simulink model "Simple_2_DPRAM_test"  (R2019b)
settings: Solver=FixedStepAuto  StartTime=0.0  StopTime=stop_time  RelTol=1e-3
InitFcn:
  | init;
StopFcn:
  | % save timeseries things as actual useful data.
values from neighbouring files (symbols this model uses):
  Addr_Bits = 4    [init.m]
  RAM_0_SEL = 0    [init.m]
  RAM_1_SEL = 1    [init.m]
  Sel_Bits = 2    [init.m]
  Ts = 1/Fs    (= 2.08333333333e-05)    [init.m]
  Ts_system = 1/Fs_system    (= 2e-08)    [init.m]
libraries: hdlsllib x7, simulink x5
settings Model: Creator=Balad  LastModifiedBy=Balad
settings SFSimCC: CustomCodeUndefinedFunction=UseInterfaceOnly

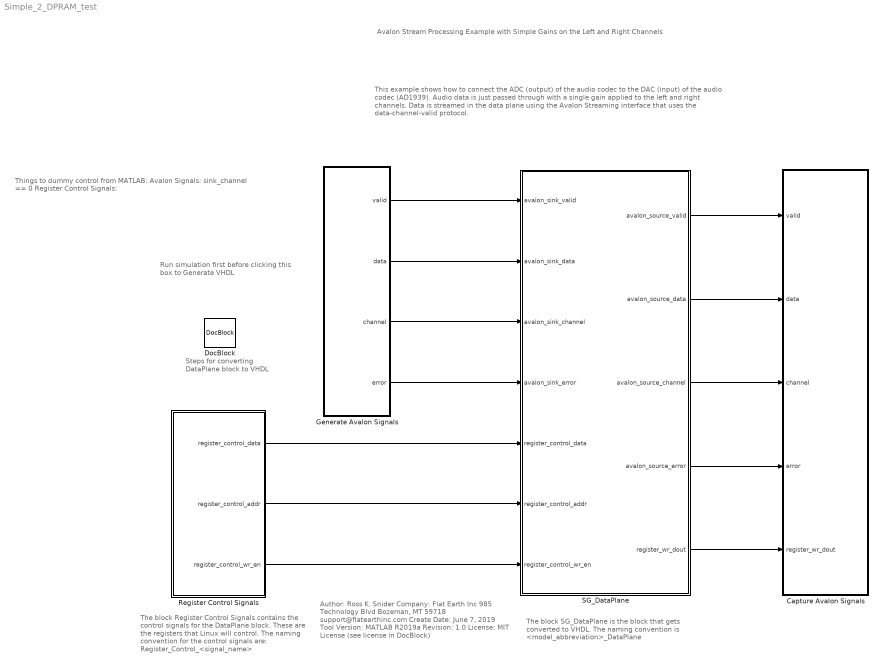
== system Simple_2_DPRAM_test ==
  note: Avalon Stream Processing Example
      | with Simple Gains on the Left and Right Channels
  note: The block SG_DataPlane is the block that gets
      | converted to VHDL. The naming convention is
      | <model_abbreviation>_DataPlane
  note: This example shows how to connect the ADC (output) of the audio codec to the DAC (input) of the audio codec (AD1939). Audio data is just passed through with a single gain applied to the left and right channels. Data is streamed in the data plane using the Avalon Streaming interface that uses the data-channel-valid protocol.
  note: The block Register Control Signals contains
      | the control signals for the DataPlane block.
      | These are the registers that Linux will control.
      | The naming convention for the control
      | signals are:  Register_Control_<signal_name>
  note: Author:          Ross K. Snider
      | Company:     Flat Earth Inc
      |                       985 Technology Blvd
      |                       Bozeman, MT 59718
      |                       support@flatearthinc.com
      | Create Date:  June 7, 2019
      | Tool Version:  MATLAB R2019a
      | Revision:        1.0
      | License:          MIT License (see license in DocBlock)
  note: Run simulation first
      | before clicking this box to
      | Generate VHDL
  note: Steps for converting
      | DataPlane block
      | to VHDL
  note: Things to dummy control from MATLAB:
      | Avalon Signals:
      | sink_channel == 0
      | Register Control Signals:
  Capture Avalon Signals : Subsystem
  DocBlock : simulink/Model-Wide Utilities/DocBlock  DocumentType=HTML
      content=|
      | <html><head></head><body>
      | Type your documentation here</body></html>
  Generate Avalon Signals : Subsystem
  Register Control Signals : Subsystem
  SG_DataPlane : Subsystem  TreatAsAtomicUnit=on
  wires:
  SG_DataPlane/2(avalon_source_data) -> Capture Avalon Signals/2(data)
  Generate Avalon Signals/1(valid) -> SG_DataPlane/1(avalon_sink_valid)
  Generate Avalon Signals/2(data) -> SG_DataPlane/2(avalon_sink_data)
  Register Control Signals/2(register_control_addr) -> SG_DataPlane/6(register_control_addr)
  SG_DataPlane/1(avalon_source_valid) -> Capture Avalon Signals/1(valid)
  SG_DataPlane/4(avalon_source_error) -> Capture Avalon Signals/4(error)
  Generate Avalon Signals/4(error) -> SG_DataPlane/4(avalon_sink_error)
  Register Control Signals/1(register_control_data) -> SG_DataPlane/5(register_control_data)
  SG_DataPlane/3(avalon_source_channel) -> Capture Avalon Signals/3(channel)
  Generate Avalon Signals/3(channel) -> SG_DataPlane/3(avalon_sink_channel)
  Register Control Signals/3("register_control_wr_en ") -> SG_DataPlane/7("register_control_wr_en ")
  SG_DataPlane/5(register_wr_dout) -> Capture Avalon Signals/5(register_wr_dout)

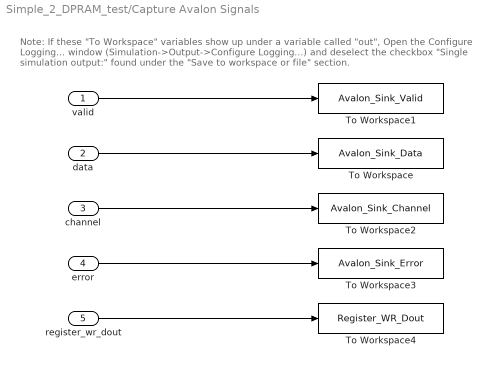
== system Simple_2_DPRAM_test/Capture Avalon Signals ==
  note: Note:  If these "To Workspace" variables show up under a variable called "out",
      | Open the Configure Logging... window (Simulation->Output->Configure Logging...)
      | and deselect the checkbox "Single simulation output:" found under the "Save to workspace or file" section.
  valid : Inport
  data : Inport  Port=2
  channel : Inport  Port=3
  error : Inport  Port=4
  register_wr_dout : Inport  Port=5
  To Workspace : ToWorkspace  VariableName=Avalon_Sink_Data  SaveFormat=Timeseries  SampleTime=-1
  To Workspace1 : ToWorkspace  VariableName=Avalon_Sink_Valid  SaveFormat=Timeseries  SampleTime=-1
  To Workspace2 : ToWorkspace  VariableName=Avalon_Sink_Channel  SaveFormat=Timeseries  SampleTime=-1
  To Workspace3 : ToWorkspace  VariableName=Avalon_Sink_Error  SaveFormat=Timeseries  SampleTime=-1
  To Workspace4 : ToWorkspace  VariableName=Register_WR_Dout  SaveFormat=Timeseries  SampleTime=-1
  wires:
  data/1 -> To Workspace/1
  valid/1 -> To Workspace1/1
  error/1 -> To Workspace3/1
  channel/1 -> To Workspace2/1
  register_wr_dout/1 -> To Workspace4/1

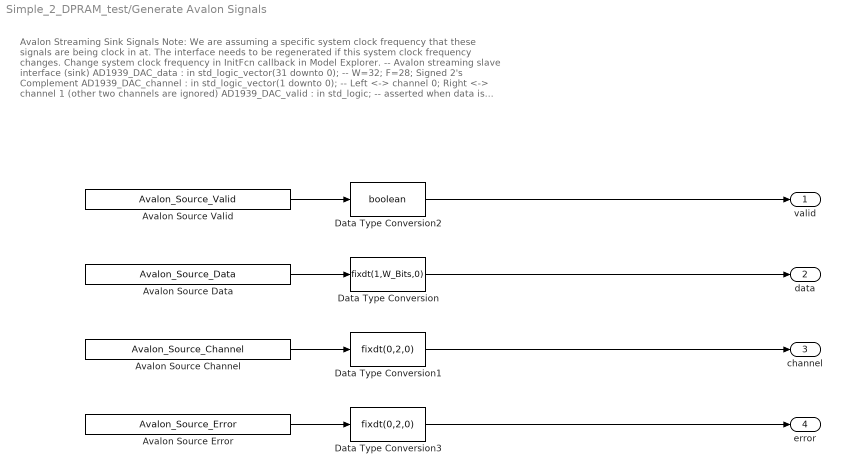
== system Simple_2_DPRAM_test/Generate Avalon Signals ==
  note: Avalon Streaming Sink Signals
      | Note: We are assuming a specific system clock frequency that these signals are being clock in at.
      | The interface needs to be regenerated if this system clock frequency changes. Change system clock frequency in InitFcn callback in Model Explorer.
      |
      | -- Avalon streaming slave interface (sink)
      | AD1939_DAC_data : in std_logic_vector(31 downto 0); -- W=32; F=28; Signed 2's Complement
      | AD1939_DAC_channel : in std_logic_vector(1 downto 0); -- Left <-> channel 0; Right <-> channel 1 (other two channels are ignored)
      | AD1939_DAC_valid : in std_logic; -- asserted when data is valid
      | AD1939_DAC_error : in std_logic_vector(1 downto 0) -- error channel is ignored, assumed to be error free at this point
      |
      | For more information on the data-channel-valid protocol, see chapter 5 in Intel's Avalon Interfaced Specification (p. 40) at https://www.intel.com/content/dam/www/programmable/us/en/pdfs/literature/manual/mnl_avalon_spec.pdf
  Avalon Source Channel : FromWorkspace  VariableName=Avalon_Source_Channel  SampleTime=Ts_system  Interpolate=off  OutputAfterFinalValue=Holding final value
  "Avalon Source Data " : FromWorkspace  VariableName=Avalon_Source_Data  SampleTime=Ts_system  Interpolate=off  OutputAfterFinalValue=Holding final value
  Avalon Source Error : FromWorkspace  VariableName=Avalon_Source_Error  SampleTime=Ts_system  Interpolate=off  OutputAfterFinalValue=Holding final value
  Avalon Source Valid : FromWorkspace  VariableName=Avalon_Source_Valid  SampleTime=Ts_system  Interpolate=off  OutputAfterFinalValue=Holding final value
  Data Type Conversion : DataTypeConversion  OutDataTypeStr=fixdt(1,W_Bits,0)
  Data Type Conversion1 : DataTypeConversion  OutDataTypeStr=fixdt(0,2,0)
  Data Type Conversion2 : DataTypeConversion  OutDataTypeStr=boolean
  Data Type Conversion3 : DataTypeConversion  OutDataTypeStr=fixdt(0,2,0)
  valid : Outport  VectorParamsAs1DForOutWhenUnconnected=off
  data : Outport  Port=2  VectorParamsAs1DForOutWhenUnconnected=off
  channel : Outport  Port=3  VectorParamsAs1DForOutWhenUnconnected=off
  error : Outport  Port=4  VectorParamsAs1DForOutWhenUnconnected=off
  wires:
  Data Type Conversion1/1 -> channel/1
  Data Type Conversion2/1 -> valid/1
  Avalon Source Error/1 -> Data Type Conversion3/1
  Data Type Conversion/1 -> data/1
  Avalon Source Valid/1 -> Data Type Conversion2/1
  Data Type Conversion3/1 -> error/1
  Avalon Source Channel/1 -> Data Type Conversion1/1
  "Avalon Source Data "/1 -> Data Type Conversion/1

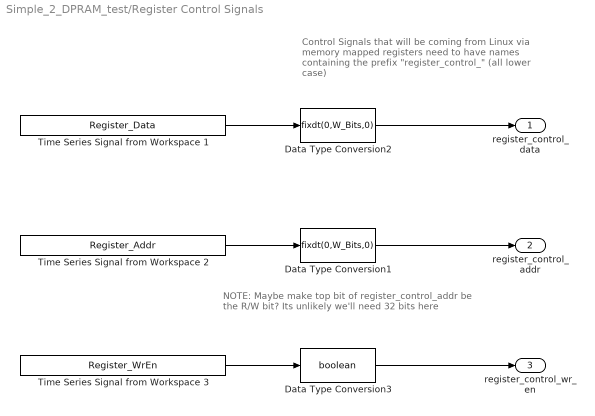
== system Simple_2_DPRAM_test/Register Control Signals ==
  note: NOTE: Maybe make top bit of register_control_addr
      | be the R/W bit? Its unlikely we'll need 32 bits here
  note: Control Signals that will be coming from Linux via
      | memory mapped registers need to have names
      | containing the prefix "register_control_"
      | (all lower case)
  Data Type Conversion1 : DataTypeConversion  OutDataTypeStr=fixdt(0,W_Bits,0)
  Data Type Conversion2 : DataTypeConversion  OutDataTypeStr=fixdt(0,W_Bits,0)
  Data Type Conversion3 : DataTypeConversion  OutDataTypeStr=boolean
  Time Series Signal from Workspace 1 : FromWorkspace  VariableName=Register_Data  OutDataTypeStr=double  SampleTime=Ts_system  OutputAfterFinalValue=Holding final value
  Time Series Signal from Workspace 2 : FromWorkspace  VariableName=Register_Addr  OutDataTypeStr=double  SampleTime=Ts_system  OutputAfterFinalValue=Holding final value
  Time Series Signal from Workspace 3 : FromWorkspace  VariableName=Register_WrEn  OutDataTypeStr=double  SampleTime=Ts_system  OutputAfterFinalValue=Holding final value
  register_control_data : Outport  VectorParamsAs1DForOutWhenUnconnected=off
  register_control_addr : Outport  Port=2  VectorParamsAs1DForOutWhenUnconnected=off
  "register_control_wr_en " : Outport  Port=3  VectorParamsAs1DForOutWhenUnconnected=off
  wires:
  Time Series Signal from Workspace 1/1 -> Data Type Conversion2/1
  Time Series Signal from Workspace 2/1 -> Data Type Conversion1/1
  Data Type Conversion2/1 -> register_control_data/1
  Data Type Conversion1/1 -> register_control_addr/1
  Data Type Conversion3/1 -> "register_control_wr_en "/1
  Time Series Signal from Workspace 3/1 -> Data Type Conversion3/1

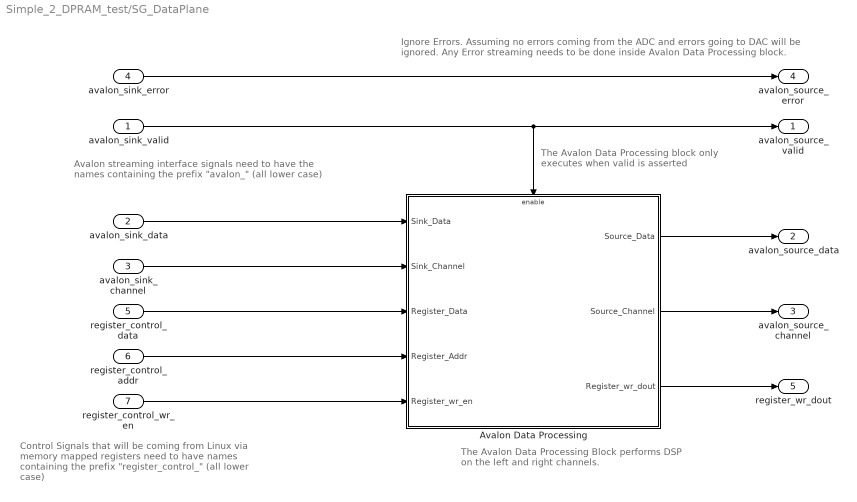
== system Simple_2_DPRAM_test/SG_DataPlane ==
  note: Control Signals that will be coming from Linux via
      | memory mapped registers need to have names
      | containing the prefix "register_control_"
      | (all lower case)
  note: The Avalon Data Processing Block
      | performs DSP on the left and right channels.
  note: The Avalon Data Processing block
      | only executes when valid is asserted
  note: Ignore Errors.
      | Assuming no errors coming from the ADC and errors going to DAC will be ignored.
      | Any Error streaming needs to be done inside Avalon Data Processing block.
  note: Avalon streaming interface signals need to have the
      | names containing the prefix "avalon_"
      | (all lower case)
  avalon_sink_valid : Inport
  avalon_sink_data : Inport  Port=2
  avalon_sink_channel : Inport  Port=3
  avalon_sink_error : Inport  Port=4
  register_control_data : Inport  Port=5
  register_control_addr : Inport  Port=6
  "register_control_wr_en " : Inport  Port=7
  Avalon Data Processing : Subsystem  TreatAsAtomicUnit=on
  avalon_source_valid : Outport  VectorParamsAs1DForOutWhenUnconnected=off
  avalon_source_data : Outport  Port=2  VectorParamsAs1DForOutWhenUnconnected=off
  avalon_source_channel : Outport  Port=3  VectorParamsAs1DForOutWhenUnconnected=off
  avalon_source_error : Outport  Port=4  VectorParamsAs1DForOutWhenUnconnected=off
  register_wr_dout : Outport  Port=5  VectorParamsAs1DForOutWhenUnconnected=off
  wires:
  avalon_sink_channel/1 -> Avalon Data Processing/2(Sink_Channel)
  avalon_sink_error/1 -> avalon_source_error/1
  Avalon Data Processing/1(Source_Data) -> avalon_source_data/1
  avalon_sink_valid/1 -> avalon_source_valid/1, Avalon Data Processing/Enable
  avalon_sink_data/1 -> Avalon Data Processing/1(Sink_Data)
  Avalon Data Processing/2(Source_Channel) -> avalon_source_channel/1
  register_control_addr/1 -> Avalon Data Processing/4(Register_Addr)
  register_control_data/1 -> Avalon Data Processing/3(Register_Data)
  "register_control_wr_en "/1 -> Avalon Data Processing/5(Register_wr_en)
  Avalon Data Processing/3(Register_wr_dout) -> register_wr_dout/1

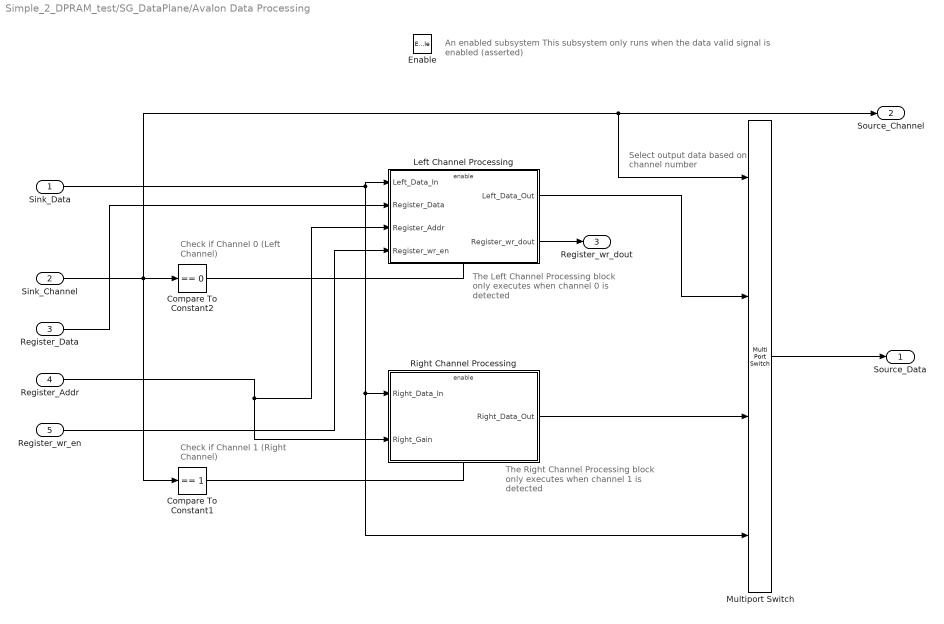
== system Simple_2_DPRAM_test/SG_DataPlane/Avalon Data Processing ==
  note: Select output data
      | based on channel number
  note: Check if Channel 0
      | (Left Channel)
  note: The Left Channel Processing block
      | only executes when channel 0
      | is detected
  note: The Right Channel Processing block
      | only executes when channel 1
      | is detected
  note: Check if Channel 1
      | (Right Channel)
  note: An enabled subsystem
      | This subsystem only runs when the data valid signal is enabled (asserted)
  Sink_Data : Inport
  Sink_Channel : Inport  Port=2
  Register_Data : Inport  Port=3
  Register_Addr : Inport  Port=4
  Register_wr_en : Inport  Port=5
  Enable : EnablePort
  Compare To Constant1 : simulink/Logic and Bit Operations/Compare To Constant  relop===  const=1  OutDataTypeStr=boolean
  Compare To Constant2 : simulink/Logic and Bit Operations/Compare To Constant  relop===  const=0  OutDataTypeStr=boolean
  Left Channel Processing : Subsystem  TreatAsAtomicUnit=on
  Multiport Switch : MultiPortSwitch  DataPortOrder=Zero-based contiguous  zeroidx=on
  Right Channel Processing : Subsystem  TreatAsAtomicUnit=on
  Source_Data : Outport  InitialOutput=0  VectorParamsAs1DForOutWhenUnconnected=off
  Source_Channel : Outport  Port=2  InitialOutput=0  VectorParamsAs1DForOutWhenUnconnected=off
  Register_wr_dout : Outport  Port=3  InitialOutput=0  VectorParamsAs1DForOutWhenUnconnected=off
  wires:
  Sink_Channel/1 -> Source_Channel/1, Multiport Switch/1, Compare To Constant1/1, Compare To Constant2/1
  Compare To Constant2/1 -> Left Channel Processing/Enable
  Compare To Constant1/1 -> Right Channel Processing/Enable
  Sink_Data/1 -> Multiport Switch/4, Right Channel Processing/1(Right_Data_In), Left Channel Processing/1(Left_Data_In)
  Left Channel Processing/1("Left_Data_Out ") -> Multiport Switch/2
  Right Channel Processing/1("Right_Data_Out ") -> Multiport Switch/3
  Multiport Switch/1 -> Source_Data/1
  Register_Data/1 -> Left Channel Processing/2(Register_Data)
  Register_Addr/1 -> Left Channel Processing/3(Register_Addr), Right Channel Processing/2(Right_Gain)
  Register_wr_en/1 -> Left Channel Processing/4(Register_wr_en)
  Left Channel Processing/2(Register_wr_dout) -> Register_wr_dout/1

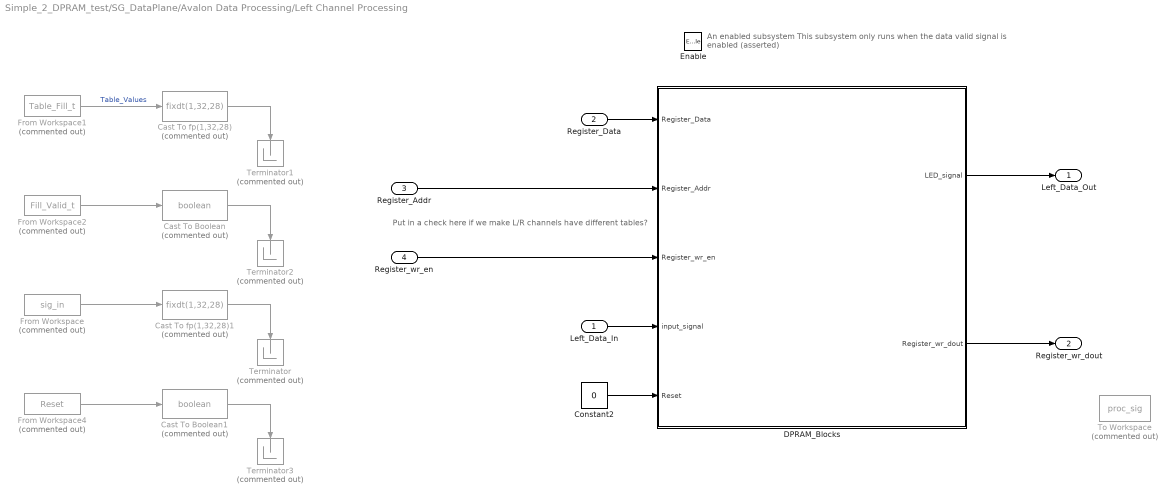
== system Simple_2_DPRAM_test/SG_DataPlane/Avalon Data Processing/Left Channel Processing ==
  note: Put in a check here if we make L/R channels have different tables?
  note: An enabled subsystem
      | This subsystem only runs when the data valid signal is enabled (asserted)
  Left_Data_In : Inport
  Register_Data : Inport  Port=2
  Register_Addr : Inport  Port=3
  Register_wr_en : Inport  Port=4
  Enable : EnablePort
  Cast To Boolean : DataTypeConversion  Commented=on  OutDataTypeStr=boolean
  Cast To Boolean1 : DataTypeConversion  Commented=on  OutDataTypeStr=boolean
  Cast To fp(1,32,28) : DataTypeConversion  Commented=on  OutDataTypeStr=fixdt(1,32,28)  RndMeth=Round
  Cast To fp(1,32,28)1 : DataTypeConversion  Commented=on  OutDataTypeStr=fixdt(1,32,28)  RndMeth=Round
  Constant2 : Constant  Value=0  OutDataTypeStr=boolean  SampleTime=-1
  DPRAM_Blocks : Subsystem
  From Workspace : FromWorkspace  Commented=on  VariableName=sig_in  SampleTime=Ts  OutputAfterFinalValue=Setting to zero
  From Workspace1 : FromWorkspace  Commented=on  VariableName=Table_Fill_t  SampleTime=Ts  Interpolate=off  OutputAfterFinalValue=Setting to zero
  From Workspace2 : FromWorkspace  Commented=on  VariableName=Fill_Valid_t  SampleTime=Ts  OutputAfterFinalValue=Setting to zero
  From Workspace4 : FromWorkspace  Commented=on  VariableName=Reset  SampleTime=Ts  Interpolate=off  OutputAfterFinalValue=Setting to zero
  Terminator{,1..3} (4 alike) : Terminator  Commented=on
  To Workspace : ToWorkspace  Commented=on  VariableName=proc_sig  SaveFormat=Timeseries  SampleTime=-1
  "Left_Data_Out " : Outport  InitialOutput=0  VectorParamsAs1DForOutWhenUnconnected=off
  Register_wr_dout : Outport  Port=2  InitialOutput=0  VectorParamsAs1DForOutWhenUnconnected=off
  wires:
  Cast To Boolean1/1 -> Terminator3/1
  Cast To Boolean/1 -> Terminator2/1
  Cast To fp(1,32,28)1/1 -> Terminator/1
  From Workspace1/1 -> Cast To fp(1,32,28)/1  "Table_Values"
  DPRAM_Blocks/1(LED_signal) -> "Left_Data_Out "/1
  From Workspace2/1 -> Cast To Boolean/1
  From Workspace/1 -> Cast To fp(1,32,28)1/1
  From Workspace4/1 -> Cast To Boolean1/1
  Cast To fp(1,32,28)/1 -> Terminator1/1
  Left_Data_In/1 -> DPRAM_Blocks/4(input_signal)
  Constant2/1 -> DPRAM_Blocks/5(Reset)
  Register_Data/1 -> DPRAM_Blocks/1(Register_Data)
  Register_Addr/1 -> DPRAM_Blocks/2(Register_Addr)
  Register_wr_en/1 -> DPRAM_Blocks/3(Register_wr_en)
  DPRAM_Blocks/2(Register_wr_dout) -> Register_wr_dout/1

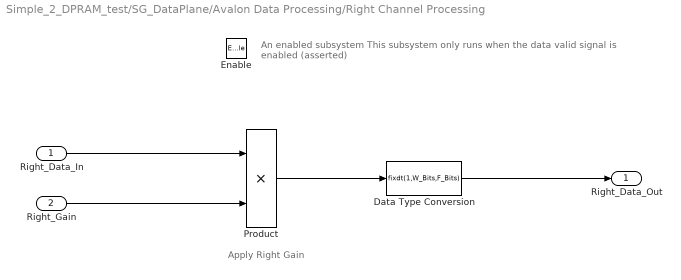
== system Simple_2_DPRAM_test/SG_DataPlane/Avalon Data Processing/Right Channel Processing ==
  note: Apply Right Gain
  note: An enabled subsystem
      | This subsystem only runs when the data valid signal is enabled (asserted)
  Right_Data_In : Inport
  Right_Gain : Inport  Port=2
  Enable : EnablePort
  Data Type Conversion : DataTypeConversion  OutDataTypeStr=fixdt(1,W_Bits,F_Bits)
  Product : Product
  "Right_Data_Out " : Outport  InitialOutput=0  VectorParamsAs1DForOutWhenUnconnected=off
  wires:
  Data Type Conversion/1 -> "Right_Data_Out "/1
  Product/1 -> Data Type Conversion/1
  Right_Data_In/1 -> Product/1
  Right_Gain/1 -> Product/2

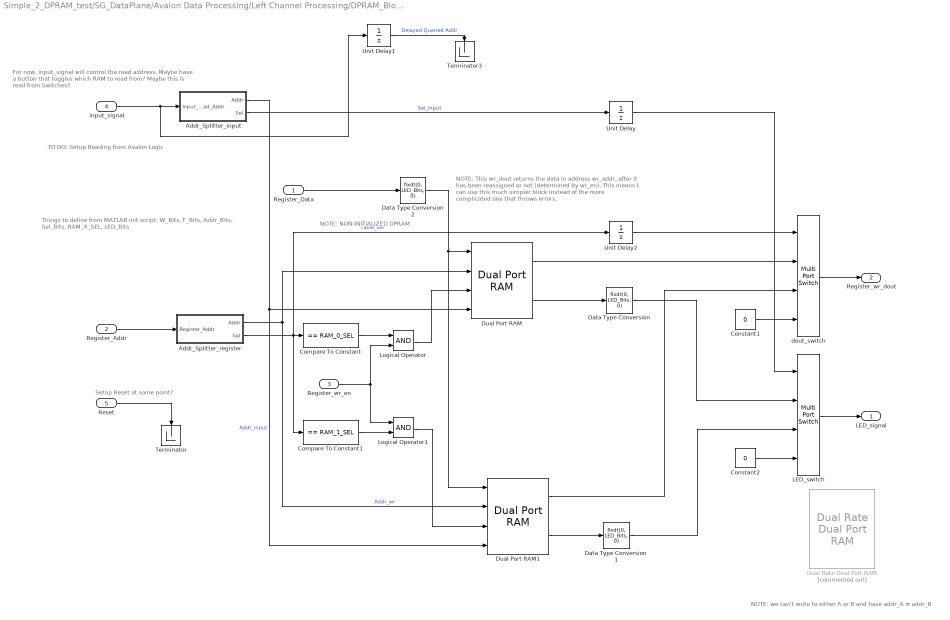
== system Simple_2_DPRAM_test/SG_DataPlane/Avalon Data Processing/Left Channel Processing/DPRAM_Blocks ==
  note: NOTE: This wr_dout returns the data in address wr_addr,
      | after it has been reassigned or not (determined by wr_en).
      | This means I can use this much simpler block instead of the
      | more complicated one that throws errors.
  note: NOTE: we can't write to either A or B and have addr_A = addr_B
  note: Things to define from MATLAB init script:
      | W_Bits, F_Bits, Addr_Bits, Sel_Bits,
      | RAM_X_SEL, LED_Bits
  note: For now, input_signal will control the read address.
      | Maybe have a button that toggles which RAM to read from?
      | Maybe this is read from Switches?
  note: TO DO: Setup Reading from Avalon Logic
  note: NOTE: NON-INITIALIZED DPRAM
  note: Setup Reset at some point?
  Register_Data : Inport
  Register_Addr : Inport  Port=2
  Register_wr_en : Inport  Port=3
  input_signal : Inport  Port=4
  Reset : Inport  Port=5
  Addr_Splitter_input : Subsystem
  Addr_Splitter_register : Subsystem
  Compare To Constant : simulink/Logic and Bit Operations/Compare To Constant  relop===  const=RAM_0_SEL  OutDataTypeStr=boolean
  Compare To Constant1 : simulink/Logic and Bit Operations/Compare To Constant  relop===  const=RAM_1_SEL  OutDataTypeStr=boolean
  Constant1 : Constant  Value=0  OutDataTypeStr=Inherit: Inherit via back propagation  SampleTime=-1
  Constant2 : Constant  Value=0  OutDataTypeStr=Inherit: Inherit via back propagation  SampleTime=-1
  Data Type Conversion : DataTypeConversion  OutDataTypeStr=fixdt(0, LED_Bits, 0)  RndMeth=Nearest
  Data Type Conversion1 : DataTypeConversion  OutDataTypeStr=fixdt(0, LED_Bits, 0)  RndMeth=Nearest
  Data Type Conversion2 : DataTypeConversion  OutDataTypeStr=fixdt(0, LED_Bits, 0)  RndMeth=Nearest
  Dual Port RAM : hdlsllib/HDL RAMs/Dual Port RAM  ram_size=Addr_Bits
      settings: SourceProductName=Simulink  SourceProductBaseCode=SL
  Dual Port RAM1 : hdlsllib/HDL RAMs/Dual Port RAM  ram_size=Addr_Bits
      settings: SourceProductName=Simulink  SourceProductBaseCode=SL
  Dual Rate Dual Port RAM : hdlsllib/HDL RAMs/Dual Rate Dual Port RAM  Commented=on  ram_size=Addr_Bits
      settings: SourceProductName=Simulink  SourceProductBaseCode=SL
  LED_switch : MultiPortSwitch  DataPortOrder=Zero-based contiguous  DataPortIndices={RAM_0_SEL, RAM_1_SEL, RAM_NULL_SEL}  DiagnosticForDefault=Warning  zeroidx=on
  Logical Operator : Logic  AllPortsSameDT=off  OutDataTypeStr=boolean
  Logical Operator1 : Logic  AllPortsSameDT=off  OutDataTypeStr=boolean
  Terminator : Terminator
  Terminator3 : Terminator
  Unit Delay : UnitDelay  SampleTime=-1  HasFrameUpgradeWarning=on
  Unit Delay1 : UnitDelay  SampleTime=-1  HasFrameUpgradeWarning=on
  Unit Delay2 : UnitDelay  SampleTime=-1  HasFrameUpgradeWarning=on
  dout_switch : MultiPortSwitch  DataPortOrder=Zero-based contiguous  DataPortIndices={RAM_0_SEL, RAM_1_SEL, RAM_NULL_SEL}  DiagnosticForDefault=Warning  zeroidx=on
  LED_signal : Outport  VectorParamsAs1DForOutWhenUnconnected=off
  Register_wr_dout : Outport  Port=2  VectorParamsAs1DForOutWhenUnconnected=off
  wires:
  Register_Addr/1 -> Addr_Splitter_register/1(Register_Addr)
  Reset/1 -> Terminator/1
  Addr_Splitter_register/2(Sel) -> Unit Delay2/1, Compare To Constant/1, Compare To Constant1/1  "Table_sel"
  Addr_Splitter_register/1(Addr) -> Dual Port RAM/2, Dual Port RAM1/2  "Addr_wr"
  Register_Data/1 -> Data Type Conversion2/1
  Dual Port RAM/1 -> dout_switch/2
  Dual Port RAM1/1 -> dout_switch/3
  Dual Port RAM/2 -> Data Type Conversion/1
  Dual Port RAM1/2 -> Data Type Conversion1/1
  input_signal/1 -> Unit Delay1/1, Addr_Splitter_input/1(Input_Read_Addr)
  Addr_Splitter_input/1(Addr) -> Dual Port RAM1/4, Dual Port RAM/4  "Addr_input"
  Data Type Conversion2/1 -> Dual Port RAM1/1, Dual Port RAM/1
  Addr_Splitter_input/2(Sel) -> Unit Delay/1  "Sel_input"
  Data Type Conversion/1 -> LED_switch/2
  Data Type Conversion1/1 -> LED_switch/3
  LED_switch/1 -> LED_signal/1
  Unit Delay/1 -> LED_switch/1
  Unit Delay1/1 -> Terminator3/1  "Delayed Queried Addr"
  Register_wr_en/1 -> Logical Operator1/1, Logical Operator/2
  Compare To Constant/1 -> Logical Operator/1
  Compare To Constant1/1 -> Logical Operator1/2
  Logical Operator1/1 -> Dual Port RAM1/3
  Logical Operator/1 -> Dual Port RAM/3
  Constant1/1 -> dout_switch/4
  dout_switch/1 -> Register_wr_dout/1
  Constant2/1 -> LED_switch/4
  Unit Delay2/1 -> dout_switch/1

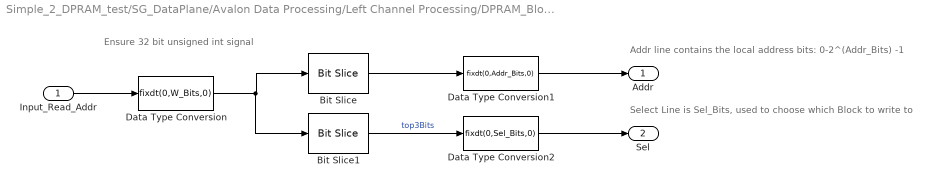
== system Simple_2_DPRAM_test/SG_DataPlane/Avalon Data Processing/Left Channel Processing/DPRAM_Blocks/Addr_Splitter_input ==
  note: Select Line is Sel_Bits, used to choose which Block to write to
  note: Addr line contains the local address bits: 0-2^(Addr_Bits) -1
  note: Ensure 32 bit unsigned int signal
  Input_Read_Addr : Inport
  Bit Slice : hdlsllib/Logic and Bit Operations/Bit Slice  lidx=Addr_Bits-1  ridx=0
      settings: SourceProductName=Simulink  SourceProductBaseCode=SL
  Bit Slice1 : hdlsllib/Logic and Bit Operations/Bit Slice  lidx=Sel_Bits+Addr_Bits-1  ridx=Addr_Bits
      settings: SourceProductName=Simulink  SourceProductBaseCode=SL
  Data Type Conversion : DataTypeConversion  OutDataTypeStr=fixdt(0,W_Bits,0)
  Data Type Conversion1 : DataTypeConversion  OutDataTypeStr=fixdt(0,Addr_Bits,0)
  Data Type Conversion2 : DataTypeConversion  OutDataTypeStr=fixdt(0,Sel_Bits,0)
  Addr : Outport  VectorParamsAs1DForOutWhenUnconnected=off
  Sel : Outport  Port=2  VectorParamsAs1DForOutWhenUnconnected=off
  wires:
  Input_Read_Addr/1 -> Data Type Conversion/1
  Data Type Conversion2/1 -> Sel/1
  Bit Slice/1 -> Data Type Conversion1/1
  Data Type Conversion/1 -> Bit Slice/1, Bit Slice1/1
  Bit Slice1/1 -> Data Type Conversion2/1  "top3Bits"
  Data Type Conversion1/1 -> Addr/1

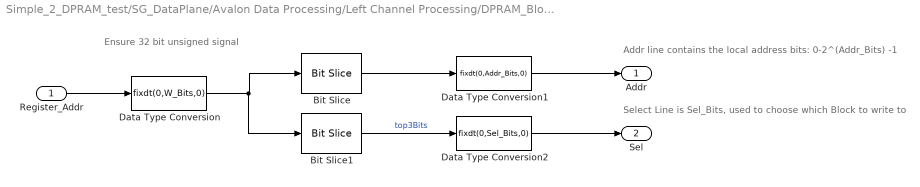
== system Simple_2_DPRAM_test/SG_DataPlane/Avalon Data Processing/Left Channel Processing/DPRAM_Blocks/Addr_Splitter_register ==
  note: Ensure 32 bit unsigned signal
  note: Addr line contains the local address bits: 0-2^(Addr_Bits) -1
  note: Select Line is Sel_Bits, used to choose which Block to write to
  Register_Addr : Inport
  Bit Slice : hdlsllib/Logic and Bit Operations/Bit Slice  lidx=Addr_Bits-1  ridx=0
      settings: SourceProductName=Simulink  SourceProductBaseCode=SL
  Bit Slice1 : hdlsllib/Logic and Bit Operations/Bit Slice  lidx=Sel_Bits+Addr_Bits-1  ridx=Addr_Bits
      settings: SourceProductName=Simulink  SourceProductBaseCode=SL
  Data Type Conversion : DataTypeConversion  OutDataTypeStr=fixdt(0,W_Bits,0)
  Data Type Conversion1 : DataTypeConversion  OutDataTypeStr=fixdt(0,Addr_Bits,0)
  Data Type Conversion2 : DataTypeConversion  OutDataTypeStr=fixdt(0,Sel_Bits,0)
  Addr : Outport  VectorParamsAs1DForOutWhenUnconnected=off
  Sel : Outport  Port=2  VectorParamsAs1DForOutWhenUnconnected=off
  wires:
  Data Type Conversion1/1 -> Addr/1
  Bit Slice1/1 -> Data Type Conversion2/1  "top3Bits"
  Data Type Conversion/1 -> Bit Slice1/1, Bit Slice/1
  Bit Slice/1 -> Data Type Conversion1/1
  Data Type Conversion2/1 -> Sel/1
  Register_Addr/1 -> Data Type Conversion/1
